simulink model "model3_algorithm"  (R2019b)
settings: Solver=VariableStepAuto  StartTime=0.0  StopTime=958  RelTol=1e-3
PreLoadFcn:
  | load SolarArrayData
undefined symbols (not defined in the file): Fs
libraries: simulink x2
settings Model: Creator=leegarth  LastModifiedBy=rdavid
settings DataIOCC: ExternalInput=[t, power]  LoadExternalInput=on

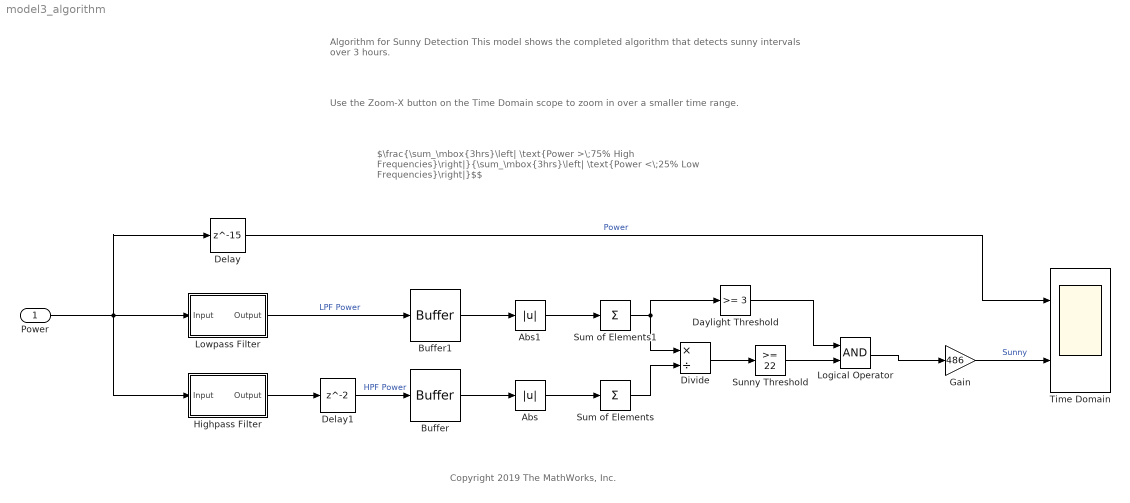
== system model3_algorithm ==
  note: $\frac{\sum_\mbox{3hrs}\left| \text{Power >\;75% High Frequencies}\right|}{\sum_\mbox{3hrs}\left| \text{Power <\;25% Low Frequencies}\right|}$$
  note: Copyright 2019 The MathWorks, Inc.
  note: Algorithm for Sunny Detection
      |
      | This model shows the completed algorithm that detects sunny intervals over 3 hours.
  note: Use the Zoom-X button on the Time Domain scope to zoom in over a smaller time range.
  Power : Inport  SampleTime=1/Fs
  Abs : Abs
  Abs1 : Abs
  Buffer : Buffer  N=12  OutputFrames=off
  Buffer1 : Buffer  N=12  OutputFrames=off
  Daylight Threshold : simulink/Logic and Bit Operations/Compare To Constant  relop=>=  const=3  OutDataTypeStr=boolean
  Delay : Delay  DelayLength=15
  Delay1 : Delay
  Divide : Product  Inputs=*/
  Gain : Gain  Gain=486
  Highpass Filter : Subsystem  Tag=FilterWizardSubSystem
      settings: ErrorFcn=dspFilterRealizedInBasicElemsAlgLoopErrFcnCallback
  Logical Operator : Logic  AllPortsSameDT=off  OutDataTypeStr=boolean
  Lowpass Filter : Subsystem  Tag=FilterWizardSubSystem
      settings: ErrorFcn=dspFilterRealizedInBasicElemsAlgLoopErrFcnCallback
  Sum of Elements : Sum  Inputs=+
  Sum of Elements1 : Sum  Inputs=+
  Sunny Threshold : simulink/Logic and Bit Operations/Compare To Constant  relop=>=  const=22  OutDataTypeStr=boolean
  Time Domain : Scope  NumInputPorts=2
  wires:
  Power/1 -> Highpass Filter/1(Input), Delay/1, Lowpass Filter/1(Input)
  Highpass Filter/1(Output) -> Delay1/1
  Delay/1 -> Time Domain/1  "Power"
  Delay1/1 -> Buffer/1  "HPF Power"
  Lowpass Filter/1(Output) -> Buffer1/1  "LPF Power"
  Buffer/1 -> Abs/1
  Buffer1/1 -> Abs1/1
  Abs/1 -> Sum of Elements/1
  Abs1/1 -> Sum of Elements1/1
  Sum of Elements/1 -> Divide/2
  Sum of Elements1/1 -> Divide/1, Daylight Threshold/1
  Divide/1 -> Sunny Threshold/1
  Gain/1 -> Time Domain/2  "Sunny"
  Daylight Threshold/1 -> Logical Operator/1
  Sunny Threshold/1 -> Logical Operator/2
  Logical Operator/1 -> Gain/1

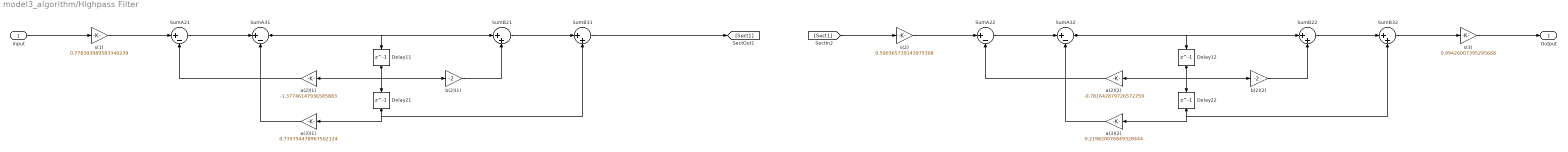
== system model3_algorithm/Highpass Filter ==
  Input : Inport
  Delay{11..12,21..22} (4 alike) : Delay  DelayLength=1  InitialCondition=0
  SumA{21..22,31..32} (4 alike) : Sum  Inputs=|+-  RndMeth=Nearest  SaturateOnIntegerOverflow=on  OutDataTypeStr=Inherit: Same as first input
  SumB{21..22,31..32} (4 alike) : Sum  Inputs=|++  RndMeth=Nearest  SaturateOnIntegerOverflow=on  OutDataTypeStr=Inherit: Same as first input
  a(2)(1) : Gain  Gain=-1.37746147936585883  ParamDataTypeStr=double  RndMeth=Nearest  SaturateOnIntegerOverflow=on  OutDataTypeStr=Inherit: Same as input
  a(2)(2) : Gain  Gain=-0.781642879726572759  ParamDataTypeStr=double  RndMeth=Nearest  SaturateOnIntegerOverflow=on  OutDataTypeStr=Inherit: Same as input
  a(3)(1) : Gain  Gain=0.735754478967502124  ParamDataTypeStr=double  RndMeth=Nearest  SaturateOnIntegerOverflow=on  OutDataTypeStr=Inherit: Same as input
  a(3)(2) : Gain  Gain=0.219820076849328444  ParamDataTypeStr=double  RndMeth=Nearest  SaturateOnIntegerOverflow=on  OutDataTypeStr=Inherit: Same as input
  b(2)(1) : Gain  Gain=-2  ParamDataTypeStr=double  RndMeth=Nearest  SaturateOnIntegerOverflow=on  OutDataTypeStr=Inherit: Same as input
  b(2)(2) : Gain  Gain=-2  ParamDataTypeStr=double  RndMeth=Nearest  SaturateOnIntegerOverflow=on  OutDataTypeStr=Inherit: Same as input
  s(1) : Gain  Gain=0.778303989583340239  ParamDataTypeStr=double  RndMeth=Nearest  SaturateOnIntegerOverflow=on  OutDataTypeStr=Inherit: Same as input
  s(2) : Gain  Gain=0.500365739143975308  ParamDataTypeStr=double  RndMeth=Nearest  SaturateOnIntegerOverflow=on  OutDataTypeStr=Inherit: Same as input
  s(3) : Gain  Gain=0.99426007395295668  ParamDataTypeStr=double  RndMeth=Nearest  SaturateOnIntegerOverflow=on  OutDataTypeStr=Inherit: Same as input
  Output : Outport
  wires:
  Input/1 -> s(1)/1
  s(1)/1 -> SumA21/1
  SumA21/1 -> SumA31/1
  SumA31/1 -> SumB21/1, Delay11/1
  SumB21/1 -> SumB31/1
  SumB31/1 -> [Sect1]
  a(2)(1)/1 -> SumA21/2
  Delay11/1 -> a(2)(1)/1, b(2)(1)/1, Delay21/1
  b(2)(1)/1 -> SumB21/2
  a(3)(1)/1 -> SumA31/2
  Delay21/1 -> a(3)(1)/1, SumB31/2
  [Sect1] -> s(2)/1
  s(2)/1 -> SumA22/1
  SumA22/1 -> SumA32/1
  SumA32/1 -> SumB22/1, Delay12/1
  SumB22/1 -> SumB32/1
  SumB32/1 -> s(3)/1
  a(2)(2)/1 -> SumA22/2
  Delay12/1 -> a(2)(2)/1, b(2)(2)/1, Delay22/1
  b(2)(2)/1 -> SumB22/2
  a(3)(2)/1 -> SumA32/2
  Delay22/1 -> a(3)(2)/1, SumB32/2
  s(3)/1 -> Output/1

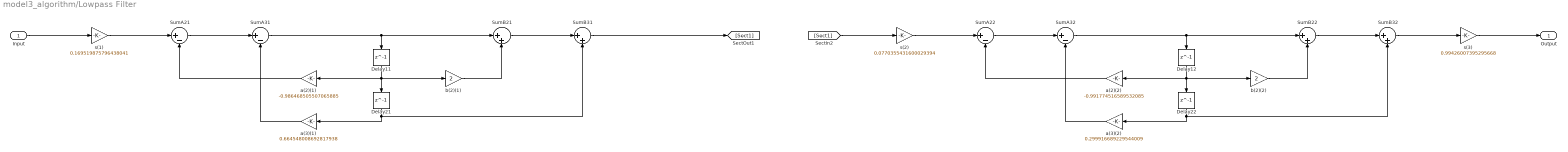
== system model3_algorithm/Lowpass Filter ==
  Input : Inport
  Delay{11..12,21..22} (4 alike) : Delay  DelayLength=1  InitialCondition=0
  SumA{21..22,31..32} (4 alike) : Sum  Inputs=|+-  RndMeth=Nearest  SaturateOnIntegerOverflow=on  OutDataTypeStr=Inherit: Same as first input
  SumB{21..22,31..32} (4 alike) : Sum  Inputs=|++  RndMeth=Nearest  SaturateOnIntegerOverflow=on  OutDataTypeStr=Inherit: Same as first input
  a(2)(1) : Gain  Gain=-0.986468505507065885  ParamDataTypeStr=double  RndMeth=Nearest  SaturateOnIntegerOverflow=on  OutDataTypeStr=Inherit: Same as input
  a(2)(2) : Gain  Gain=-0.991774516589532085  ParamDataTypeStr=double  RndMeth=Nearest  SaturateOnIntegerOverflow=on  OutDataTypeStr=Inherit: Same as input
  a(3)(1) : Gain  Gain=0.664548008692817938  ParamDataTypeStr=double  RndMeth=Nearest  SaturateOnIntegerOverflow=on  OutDataTypeStr=Inherit: Same as input
  a(3)(2) : Gain  Gain=0.299916689229544009  ParamDataTypeStr=double  RndMeth=Nearest  SaturateOnIntegerOverflow=on  OutDataTypeStr=Inherit: Same as input
  b(2)(1) : Gain  Gain=2  ParamDataTypeStr=double  RndMeth=Nearest  SaturateOnIntegerOverflow=on  OutDataTypeStr=Inherit: Same as input
  b(2)(2) : Gain  Gain=2  ParamDataTypeStr=double  RndMeth=Nearest  SaturateOnIntegerOverflow=on  OutDataTypeStr=Inherit: Same as input
  s(1) : Gain  Gain=0.169519875796438041  ParamDataTypeStr=double  RndMeth=Nearest  SaturateOnIntegerOverflow=on  OutDataTypeStr=Inherit: Same as input
  s(2) : Gain  Gain=0.0770355431600029394  ParamDataTypeStr=double  RndMeth=Nearest  SaturateOnIntegerOverflow=on  OutDataTypeStr=Inherit: Same as input
  s(3) : Gain  Gain=0.99426007395295668  ParamDataTypeStr=double  RndMeth=Nearest  SaturateOnIntegerOverflow=on  OutDataTypeStr=Inherit: Same as input
  Output : Outport
  wires:
  Input/1 -> s(1)/1
  s(1)/1 -> SumA21/1
  SumA21/1 -> SumA31/1
  SumA31/1 -> SumB21/1, Delay11/1
  SumB21/1 -> SumB31/1
  SumB31/1 -> [Sect1]
  a(2)(1)/1 -> SumA21/2
  Delay11/1 -> a(2)(1)/1, b(2)(1)/1, Delay21/1
  b(2)(1)/1 -> SumB21/2
  a(3)(1)/1 -> SumA31/2
  Delay21/1 -> a(3)(1)/1, SumB31/2
  [Sect1] -> s(2)/1
  s(2)/1 -> SumA22/1
  SumA22/1 -> SumA32/1
  SumA32/1 -> SumB22/1, Delay12/1
  SumB22/1 -> SumB32/1
  SumB32/1 -> s(3)/1
  a(2)(2)/1 -> SumA22/2
  Delay12/1 -> a(2)(2)/1, b(2)(2)/1, Delay22/1
  b(2)(2)/1 -> SumB22/2
  a(3)(2)/1 -> SumA32/2
  Delay22/1 -> a(3)(2)/1, SumB32/2
  s(3)/1 -> Output/1
